simulink model "Cuckoo"  (R2020a)
settings: Solver=VariableStepAuto  StartTime=0.0  StopTime=2  MaxStep=1e-4  RelTol=1e-3
libraries: powerlib x16, re_lib x5, powerlib_meascontrol x1
settings Model: Creator=Mahesh Krishna  LastModifiedBy=vankurua
settings DataIOCC: ReturnWorkspaceOutputs=off
settings OptimizationCC: LifeSpan=inf
settings DebuggingCC: ArithmeticOperatorsInVariantConditions=warning
settings SFSimCC: SimUseLocalCustomCode=off  CustomCodeUndefinedFunction=UseInterfaceOnly
settings RTWCC: RTWUseLocalCustomCode=off
settings CodeAppCC: StateflowObjectComments=on
settings SimscapeCC: SimscapeNormalizeSystem=off

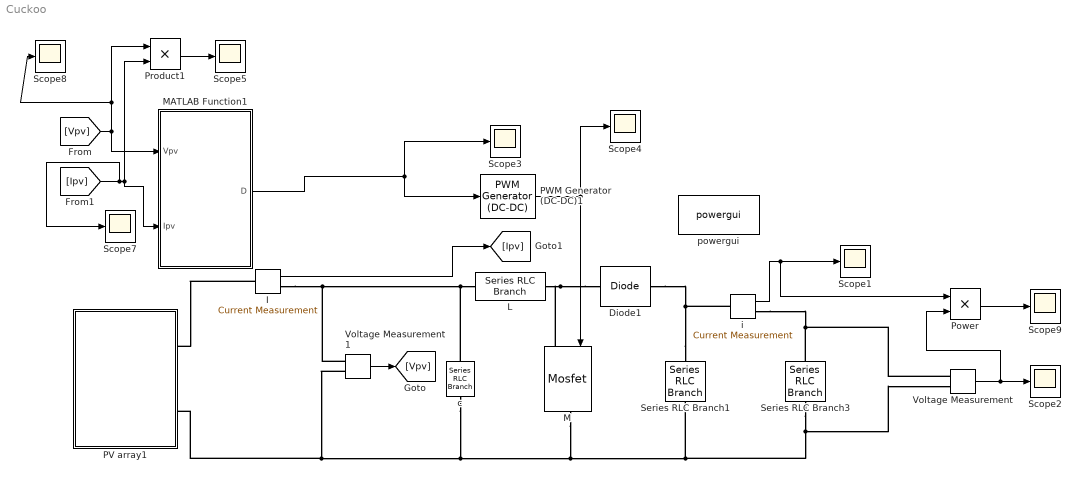
== system Cuckoo ==
  Diode1 : powerlib/Power Electronics/Diode  Ron=1e-3  Lon=0  Vf=0  IC=0  UseSnubber=off  Rs=inf  Cs=inf  Measurements=off
  I : powerlib/Measurements/Current Measurement  PhasorSimulation=off  OutputType=Magnitude  PSBequivalent=0
  L : powerlib/Elements/Series RLC Branch  LConnTagsString=__new0  RConnTagsString=__new0  BranchType=L  Resistance=1e-3  Inductance=5e-3  SetiL0=off  InitialCurrent=0  Capacitance=1e-6  Setx0=off  InitialVoltage=0  Measurements=None
  M : powerlib/Power Electronics/Mosfet  Ron=1e-3  Lon=0  Rd=1e-3  Vfd=0  IC=0  Rs=inf  Cs=inf  Measurements=off
  MATLAB Function1 : MATLAB Function  TreatAsAtomicUnit=on
  PV array1 : Subsystem
  PWM Generator (DC-DC)1 : powerlib_meascontrol/Pulse & Signal Generators/PWM Generator (DC-DC)  Fsw=20000  Ts=0
  Power : Product
  Product1 : Product
  Scope{1..5,7..9} (8 alike) : Scope
  Series RLC Branch1 : powerlib/Elements/Series RLC Branch  LConnTagsString=__new0  RConnTagsString=__new0  BranchType=C  Resistance=1e-4  Inductance=200e-6  SetiL0=off  InitialCurrent=0  Capacitance=22e-6  Setx0=off  InitialVoltage=40  Measurements=None
  Series RLC Branch3 : powerlib/Elements/Series RLC Branch  LConnTagsString=__new0  RConnTagsString=__new0  BranchType=R  Resistance=100  Inductance=200e-6  SetiL0=off  InitialCurrent=0  Capacitance=1000e-6  Setx0=off  InitialVoltage=40  Measurements=None
  Voltage Measurement : powerlib/Measurements/Voltage Measurement  PhasorSimulation=off  OutputType=Magnitude  PSBequivalent=0
  Voltage Measurement1 : powerlib/Measurements/Voltage Measurement  PhasorSimulation=off  OutputType=Magnitude  PSBequivalent=0
  c : powerlib/Elements/Series RLC Branch  LConnTagsString=__new0  RConnTagsString=__new0  BranchType=C  Resistance=1e-3  Inductance=250e-6  SetiL0=off  InitialCurrent=0  Capacitance=2.2e-6  Setx0=off  InitialVoltage=0  Measurements=None
  i : powerlib/Measurements/Current Measurement  PhasorSimulation=off  OutputType=Magnitude  PSBequivalent=0
  powergui : powerlib/powergui  Priority=1  SimulationMode=Continuous  SampleTime=50e-6  frequency=60  Iterations=50  frequencyindice=0  Pbase=100e6  ErrMax=1e-4  UnitsV=kV  UnitsW=MW  buscounter=0  FunctionMessages=off  echomessages=off  EnableUseOfTLC=off  CurrentSourceSwitches=off  DisableSnubberDevices=off  DisableRonSwitches=off  DisableVfSwitches=off  DisplayEquations=off  AutomaticDiscreteSolvers=off  SolverType=Tustin/Backward Euler (TBE)  Interpol=off  ExternalGateDelay=off  methode=off  Ts=100  x0status=blocks  SPID=on  SwTol=0  HookPort=off  NonlinearTolerance=1e-4  nMaxIteration=100  ContinueOnMaxIteration=off  RestoreLinks=warning  ResistiveCurrentMeasurement=off  Frange=[0:2:500]  Ylog=off  Xlog=on  ShowGrid=off  save=off  variable=ZData  structure=0  ZoomFFT=off  StartTime=0.0  cycles=1  DisplayStyle=1  fundamental=60  FreqAxis=off  MaxFrequency=1000  frequencyindicesteady=1  RmsSteady=1  display=off
  wires:
  I/1 -> [Ipv]
  [Ipv] -> Scope7/1, MATLAB Function1/2(Ipv), Product1/2
  Voltage Measurement/1 -> Power/2, Scope2/1
  PWM Generator (DC-DC)1/1 -> Scope4/1, M/1
  i/1 -> Power/1, Scope1/1
  Voltage Measurement1/1 -> [Vpv]
  [Vpv] -> MATLAB Function1/1(Vpv), Scope8/1, Product1/1
  Product1/1 -> Scope5/1
  Power/1 -> Scope9/1
  MATLAB Function1/1(D) -> Scope3/1, PWM Generator (DC-DC)1/1
  connections:
  i/RConn1 -- Series RLC Branch3/LConn1 -- Voltage Measurement/LConn1
  Series RLC Branch1/RConn1 -- Series RLC Branch3/RConn1 -- Voltage Measurement/LConn2 -- Voltage Measurement1/LConn2 -- PV array1/RConn2 -- c/RConn1 -- M/RConn1
  Series RLC Branch1/LConn1 -- Diode1/RConn1 -- i/LConn1
  I/LConn1 -- PV array1/RConn1
  Diode1/LConn1 -- M/LConn1 -- L/RConn1
  I/RConn1 -- Voltage Measurement1/LConn1 -- c/LConn1 -- L/LConn1

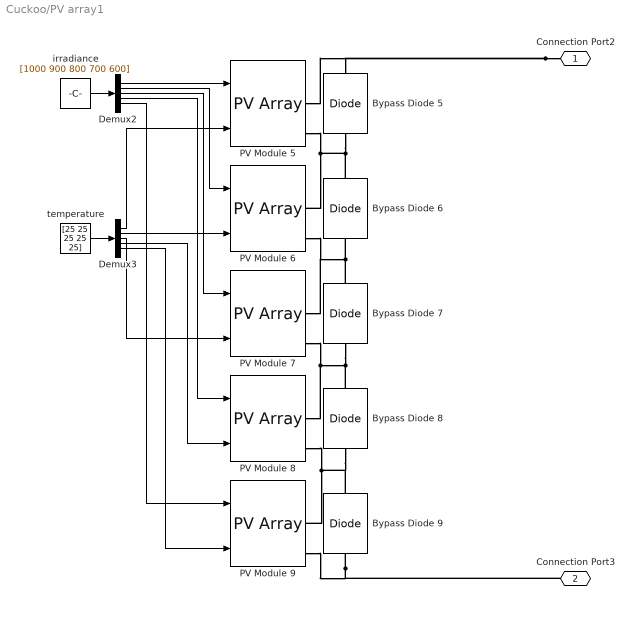
== system Cuckoo/PV array1 ==
  Bypass Diode {5..9} (5 alike) : powerlib/Power Electronics/Diode  Ron=0.001  Lon=0  Vf=0.8  IC=0  UseSnubber=off  Rs=500  Cs=250e-9  Measurements=off
  Demux2 : Demux  Outputs=5
  Demux3 : Demux  Outputs=5
  PV Module {5..9} (5 alike) : re_lib/Solar/PV Array  Npar=1  Nser=1  PlotType=array @ 1000 W/m2 & specified temperatures  S_vec="[ 1000  500  100 ]"  Temp_C_vec="[ 45 25  ]"  ModuleName=ET Solar Industry ET-P654200WW  PlotWhenSelected=off  Pm=200.2656  Ncell=54  Voc=32.72  Isc=7.86  Vm=27.21  Im=7.36  beta_Voc_pc=-0.35691  alpha_Isc_pc=0.050102  beta_Voc=-0.11678  alpha_Isc=0.003938  IL=7.8912  I0=2.3497e-10  nI=0.974  Rsh=176.8846  Rs=0.19523  RobustModel=off  RobustCellTemperature=25  BAL=off  Tc=1e-6  Tfilter=5e-5
  irradiance : Constant  Value=[1000 900 800 700 600]
  temperature : Constant  Value=[25 25 25 25 25]
  Connection Port2 : PMIOPort  Side=Right
  Connection Port3 : PMIOPort  Port=2  Side=Right
  wires:
  Demux2/1 -> PV Module 5/1
  Demux3/4 -> PV Module 8/2
  Demux3/1 -> PV Module 5/2
  Demux3/3 -> PV Module 7/2
  Demux2/5 -> PV Module 9/1
  Demux2/4 -> PV Module 8/1
  Demux2/3 -> PV Module 7/1
  Demux3/5 -> PV Module 9/2
  irradiance/1 -> Demux2/1
  Demux2/2 -> PV Module 6/1
  temperature/1 -> Demux3/1
  Demux3/2 -> PV Module 6/2
  connections:
  Bypass Diode 6/RConn1 -- Bypass Diode 5/LConn1 -- PV Module 5/RConn2 -- PV Module 6/RConn1
  Connection Port2/RConn1 -- PV Module 5/RConn1 -- Bypass Diode 5/RConn1
  Bypass Diode 9/LConn1 -- Connection Port3/RConn1 -- PV Module 9/RConn2
  Bypass Diode 7/RConn1 -- Bypass Diode 6/LConn1 -- PV Module 7/RConn1 -- PV Module 6/RConn2
  PV Module 8/RConn2 -- PV Module 9/RConn1 -- Bypass Diode 8/LConn1 -- Bypass Diode 9/RConn1
  PV Module 7/RConn2 -- PV Module 8/RConn1 -- Bypass Diode 7/LConn1 -- Bypass Diode 8/RConn1

== matlab function Cuckoo/MATLAB Function1 ==
  settings: updateMethod=DISCRETE  sampleTime=1e-4
  data: Vpv input; D output; Ipv input
function D = Cuckoo(Vpv,Ipv)
%#codegen
persistent u;
persistent dcurrent;
persistent p;
persistent dc;
persistent dbest;
persistent counter;
persistent iworst;
persistent discover;
if(isempty(discover))
    discover=0;
end
if(isempty(counter))
    counter=0;
end
if(isempty(dcurrent))
    dcurrent=0.5;
end
if(isempty(iworst))
    iworst=0;
end



if(isempty(dbest))
    dbest=0;
end
if(isempty(p))
    p=zeros(4,1);
end
if(isempty(u))
    u=0;
end
if(isempty(dc))
    dc=zeros(4,1);
    dc(1)=0;
    dc(2)=0.3;
    dc(3)=0.5;
    dc(4)=0.9;
end
if(counter>=1 && counter<150)
    D=dcurrent;
    counter=counter+1;
    return;
end
counter=0;

if(u>=1 && u<=4)
    p(u)=Vpv*Ipv;
end
u=u+1;
if(u==7)
    u=1;
end
if(u==1)
    D=dc(u);
    dcurrent=D;
    counter=1;
    return;
elseif(u==2)
    D=dc(u);
    dcurrent=D;
    counter=1;
    return;
elseif(u==3)
    D=dc(u);
    dcurrent=D;
    counter=1;
    return;
elseif(u==4)
    D=dc(u);
    dcurrent=D;
    counter=1;
    return;
elseif(u==5 || u==6 )
    if(u==5)
        if(rand(1)>0.25)
            discover=1;
            [m,i]=max(p)
            dbest=dc(i);
            %determine the worst nest
            [m,iworst]=min(p);
            %build new nest
            %dc(iworst)=dbest;
            dc(iworst)=levyflight(dbest,dc(iworst));
            %dc(iworst)=withinlimits(dc(iworst));
            D=dc(iworst);
            dcurrent=D;
            counter=1;
            return;
        else
            u=u+1;
            [m,i]=max(p)
            dbest=dc(i);
            D=dbest;
            dcurrent=D;
            counter=1;
            dc(1)=levyflight(dbest,dc(1))
            % dc(1)=withinlimits(dc(1))
            dc(2)=levyflight(dbest,dc(2))
            %dc(2)=withinlimits(dc(2))
            dc(3)=levyflight(dbest,dc(3))
            % dc(3)=withinlimits(dc(3))
            dc(4)=levyflight(dbest,dc(4))
            % dc(4)=withinlimits(dc(4))
            return;
        end
        
    else
        %calculate new power of new nest
        p(iworst)=Vpv*Ipv;
        %determine the best nest
        [m,i]=max(p);
        dbest=dc(i);
        D=dbest;
        dcurrent=D;
        counter=1;
        
        dc(1)=levyflight(dbest,dc(1))
        % dc(1)=withinlimits(dc(1))
        dc(2)=levyflight(dbest,dc(2))
        %dc(2)=withinlimits(dc(2))
        dc(3)=levyflight(dbest,dc(3))
        % dc(3)=withinlimits(dc(3))
        dc(4)=levyflight(dbest,dc(4))
        % dc(4)=withinlimits(dc(4))
        discover=0;
        return;
    end
    
else
    u
    y='hello'
    D=0.1
    
end


end
function dfinal=levyflight(dbest,d)
beta=3/2;
kcoeff=0.8;
sigmau=(gamma(1+beta)*sin(pi*beta/2)/(gamma((1+beta)/2)*beta*2^((beta-1)/2)))^(1/beta);
sigmav=1;
u=normrnd(0,(sigmau)^2);
v=normrnd(0,(sigmav)^2);
dup=d+(kcoeff*(abs(u)/((abs(v))^(1/beta)))*(dbest-d));


if(dup>1)
    dfinal=1;
elseif(dup<0)
    dfinal=0;
else
    dfinal=dup;
end
end
